simulink model "testI2t"  (R2016b)
settings: Solver=FixedStepAuto  StartTime=0.0  StopTime=500  FixedStep=0.001  RelTol=1e-3
libraries: I2t x1
settings Model: Creator=Taeke  LastModifiedBy=Marc

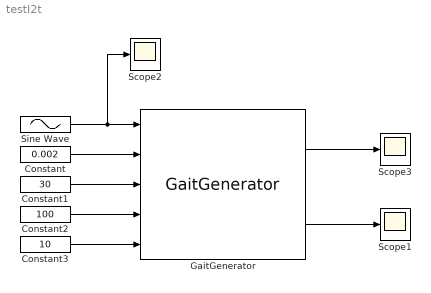
== system testI2t ==
  Constant : Constant  Value=0.002
  Constant1 : Constant  Value=30
  Constant2 : Constant  Value=100
  Constant3 : Constant  Value=10
  GaitGenerator : I2t/GaitGenerator
  Scope1 : Scope
  Scope2 : Scope
  Scope3 : Scope
  Sine Wave : Sin  Amplitude=20  Bias=20  Frequency=0.1/(2*pi)  SampleTime=0.002
  wires:
  Sine Wave/1 -> GaitGenerator/1, Scope2/1
  GaitGenerator/1 -> Scope3/1
  GaitGenerator/2 -> Scope1/1
  Constant/1 -> GaitGenerator/2
  Constant3/1 -> GaitGenerator/5
  Constant2/1 -> GaitGenerator/4
  Constant1/1 -> GaitGenerator/3
